simulink model "PID_Pendulum"  (R2018a)
settings: Solver=ode5  StartTime=0.0  StopTime=300  FixedStep=0.1  RelTol=1e-3
undefined symbols (not defined in the file): sigbuilder_block
libraries: fuzblock x1
settings Model: Creator=ACER  LastModifiedBy=DELL

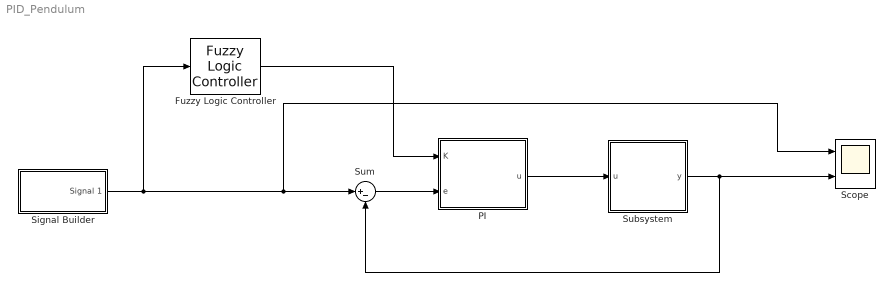
== system PID_Pendulum ==
  Fuzzy Logic Controller : fuzblock/Fuzzy Logic  Controller  FIS='fuzzy_pid.fis'  OutputSampleNumber=101  DataType=double  FuzzifiedInputs=off  RuleFiringStrengths=off  RuleOutputs=off  AggregatedOutputs=off  SimulateUsing=Interpreted execution  OutOfRangeInputValueMessage=warning  NoRuleFiredMessage=warning  EmptyOutputFuzzySetMessage=warning
  PI : Subsystem
  Scope : Scope  NumInputPorts=2
  Signal Builder : Subsystem  Tag=STV Subsys  LoadFcn=sigbuilder_block('load');  StartFcn=sigbuilder_block('start');  StopFcn=sigbuilder_block('stop');  ClipboardFcn=sigbuilder_block('clipboard');  mask(Sigbuilder block){tuvar=[0:10]}
      mask help: Simulink:masks:SigbuilderBlock_MD
      mask init:
      | if ~strcmp(get_param(bdroot(gcbh),'SimulationStatus'),'stopped') tuvar = sigbuilder_block('maskInit'); end
      settings: CopyFcn=sigbuilder_block('copy');  DeleteFcn=sigbuilder_block('delete');  ModelCloseFcn=sigbuilder_block('modelClose');  PreSaveFcn=sigbuilder_block('preSave');  PauseFcn=sigbuilder_block('pause');  ContinueFcn=sigbuilder_block('continue');  NameChangeFcn=sigbuilder_block('namechange');  OpenFcn=sigbuilder_block('open',[369.6 76.8 550.8 400.2 ]);  CloseFcn=sigbuilder_block('close');
      mask Display: plot(0, 0, 100, 100,[2, 2, 32, 32, 2], [68, 8, 8, 68, 68],[32, 2], [38, 38], [32, 19, 2],[53, 60, 44], [32, 17, 17, 2],[16, 16, 31, 31]);txt = getActiveGroup(gcbh);text(2, 100, txt,'verticalAlignment', 'top');
  Subsystem : Subsystem  mask{b=1.5, C=0.8, K=50, g=981, Rmax=20, Rmin=10, Ymax=100}
  Sum : Sum  Inputs=|+-
  wires:
  Subsystem/1(y) -> Sum/2, Scope/2
  Fuzzy Logic Controller/1 -> PI/1(K)
  PI/1(u) -> Subsystem/1(u)
  Sum/1 -> PI/2(e)
  Signal Builder/1(Signal 1) -> Fuzzy Logic Controller/1, Scope/1, Sum/1

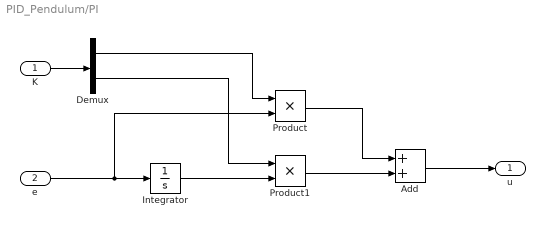
== system PID_Pendulum/PI ==
  K : Inport
  e : Inport  Port=2
  Add : Sum  Inputs=2
  Demux : Demux  Outputs=2
  Integrator : Integrator
  Product : Product
  Product1 : Product
  u : Outport
  wires:
  K/1 -> Demux/1
  Demux/1 -> Product/1
  e/1 -> Product/2, Integrator/1
  Product/1 -> Add/1
  Product1/1 -> Add/2
  Add/1 -> u/1
  Integrator/1 -> Product1/2
  Demux/2 -> Product1/1

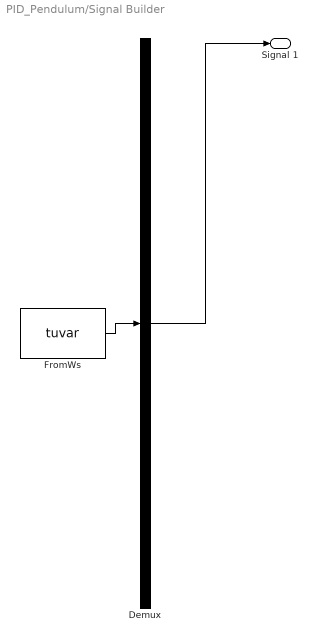
== system PID_Pendulum/Signal Builder ==
  Demux : Demux  Tag=STV Demux  Outputs=1
  FromWs : FromWorkspace  Tag=STV FromWs  VariableName=tuvar  SampleTime=0
      SigBuilderData=|
      | common.afterFinalStr = 'Extrapolate'
      | common.sampleTime = 0
      | dataSet.timeRange = [0 300]
      | dataSet.name = 'Group 1'
      | sbobj.Groups.Name = 'Group 1'
      | sbobj.Groups.Signals.Name = 'Signal 1'
      | sbobj.Groups.Signals.XData = [0 50.5 50.5 100.5 100.5 150.5 150.5 200.5 200.5 250.5 250.5 300]
      | sbobj.Groups.Signals.YData = [90 90 50 50 10 10 70 70 30 30 89.5 89.5]
      | sbobj.Groups.TimeRange = [0 300]
  Signal 1 : Outport  Tag=STV Outport
  wires:
  Demux/1 -> Signal 1/1
  FromWs/1 -> Demux/1

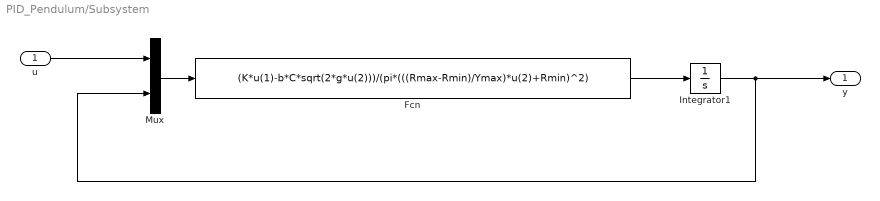
== system PID_Pendulum/Subsystem ==
  u : Inport
  Fcn : Fcn  Expr=(K*u(1)-b*C*sqrt(2*g*u(2)))/(pi*(((Rmax-Rmin)/Ymax)*u(2)+Rmin)^2)
  Integrator1 : Integrator
  Mux : Mux  Inputs=2
  y : Outport
  wires:
  Integrator1/1 -> y/1, Mux/2
  Fcn/1 -> Integrator1/1
  Mux/1 -> Fcn/1
  u/1 -> Mux/1
